simulink model "rev0BB"  (R2017b)
settings: Solver=FixedStepDiscrete  StartTime=0  StopTime=(((preLen+100+dataLenSymbols)*1+pad_first*3)*basePer)  RelTol=1e-3
values from neighbouring files (symbols this model uses):
  ack_stf_len_symbols = length(x_ACK_STF)    [rev0BB_setup.m]
  agc_delay_lag = 32    [rev0BB_setup.m]
  agc_detector_coef = ones(1,agc_detector_taps)./agc_detector_taps    [rev0BB_setup.m]
  agc_on = true    [rev0BB_startup.m]
  agc_sat_low = -agcSaturation    (= -12)    [rev0BB_setup.m]
  agc_sat_up = agcSaturation    (= 12)    [rev0BB_setup.m]
  agcDesired = 0    [rev0BB_setup.m]
  agcExpDomain = agcSaturation    (= 12)    [rev0BB_setup.m]
  agcExpResolution = 2^-5    (= 0.03125)    [rev0BB_setup.m]
  agcPwrAvgNum = 128    [rev0BB_setup.m]
  agcSaturation = 12    [rev0BB_setup.m]
  agcSettleThresh = 0.65    [rev0BB_setup.m]
  agcStep = 2^-8    (= 0.00390625)    [rev0BB_setup.m]
  atanDomain = 5    [rev0BB_setup.m]
  atanDomainTiming = 256    [rev0BB_setup.m]
  atanResolution = 2^-9    (= 0.001953125)    [rev0BB_setup.m]
  atanResolutionTiming = 2^-5    (= 0.03125)    [rev0BB_setup.m]
  averaging_num = ones(1, averaging_samples)    [rev0BB_setup.m]
  averaging_samples = 128    [rev0BB_setup.m]
  awgnSeed = abs(dBSnrRange(dBSnrInd)*1000+trial+10000000)    [plotBer.m]    (also in rev0BB_startup.m = 67)
  basePer = 1/baseFreq    (= 5e-08)    [rev0BB_setup.m]
  bitsPerSymbolHeader = log2(radixHeader)    [rev0BB_setup.m]
  bitsPerSymbolMax = log2(radixMax)    [rev0BB_setup.m]
  cal_sig_i_mult = 1.0    (= 1)    [rev0BB_startup.m]
  cal_sig_i_offset = 0.0    (= 0)    [rev0BB_startup.m]
  cal_sig_q_mult = 1.0    (= 1)    [rev0BB_startup.m]
  cal_sig_q_offset = 0.0    (= 0)    [rev0BB_startup.m]
  cefEarlyWarning = 256    [rev0BB_setup.m]
  cefLen = length(x_CEF)    [rev0BB_setup.m]
  channelFIR = zeros(1, round(maxSampleDelay)+1)    [rev0BB_startup.m]
  coarseCFOAdaptDelay = 1    [rev0BB_setup.m]
  cr_i = 0.020    (= 0.02)    [rev0BB_setup.m]
  cr_i_preamp = 2^-9    (= 0.001953125)    [rev0BB_setup.m]
  cr_int1_sat_low = -cr_integrator1_saturation    (= -0.6)    [rev0BB_setup.m]
  cr_int1_sat_up = cr_integrator1_saturation    (= 0.6)    [rev0BB_setup.m]
  cr_integrator1_decay = 1    [rev0BB_setup.m]
  cr_integrator1_saturation = 0.6    [rev0BB_setup.m]
  cr_mult_pipeline = 0    [rev0BB_setup.m]
  cr_p = 0.015    [rev0BB_setup.m]
  cr_sat2_low = -cr_saturation2    (= -0.6)    [rev0BB_setup.m]
  cr_sat2_up = cr_saturation2    (= 0.6)    [rev0BB_setup.m]
  cr_smooth_num = (1/cr_smooth_samples).*ones(1, cr_smooth_samples)    [rev0BB_setup.m]
  D_128 = [ 1,  8,  2,  4, 16, 32, 64]    [golay.m]    (also in rev0BB_setup.m)
  D_32 = [ 1,  4,  8,  2, 16]    [golay.m]    (also in rev0BB_setup.m)
  dataLenSymbols = header_len_bytes*8/bitsPerSymbolHeader + frame_len_bytes*8/bitsPerSymbol    [rev0BB_setup.m]
  default_channel = 3    [rev0BB_setup.m]
  dmm_coefs = ones(1,dmm_samples)./dmm_samples    [rev0BB_setup.m]
  dst_field_len = 8    [rev0BB_setup.m]
  expDomain = 3.3    [rev0BB_setup.m]
  expResolution = 2^-5    (= 0.03125)    [rev0BB_setup.m]
  expTol = .1    (= 0.1)    [rev0BB_setup.m]
  flush_delay = regular_pipeline*2+mult_pipeline+4    (= 4)    [rev0BB_setup.m]
  frac_lut_domain = 256    [rev0BB_setup.m]
  frac_lut_domain_cr = 64    [rev0BB_setup.m]
  frac_lut_range_max = 512    [rev0BB_setup.m]
  frac_lut_range_max_coarse_cfo = 127    [rev0BB_setup.m]
  frac_lut_range_max_cr = 127    [rev0BB_setup.m]
  frac_lut_range_min = -frac_lut_range_max    (= -512)    [rev0BB_setup.m]
  frac_lut_range_min_coarse_cfo = -frac_lut_range_max_coarse_cfo    (= -127)    [rev0BB_setup.m]
  frac_lut_range_min_cr = -frac_lut_range_max_cr    (= -127)    [rev0BB_setup.m]
  frac_lut_table_breaks = -frac_lut_domain:frac_lut_res:(frac_lut_domain-1)    [rev0BB_setup.m]
  frac_lut_table_breaks_coarse_cfo = -frac_lut_domain_coarse_cfo:frac_lut_res_coarse_cfo:(frac_lut_domain_coarse_cfo-1)    [rev0BB_setup.m]
  frac_lut_table_breaks_cr = -frac_lut_domain_cr:frac_lut_res_cr:(frac_lut_domain_cr-1)    [rev0BB_setup.m]
  frac_lut_table_data = 1./frac_lut_table_breaks    [rev0BB_setup.m]
  frac_lut_table_data_coarse_cfo = 1./frac_lut_table_breaks_coarse_cfo    [rev0BB_setup.m]
  frac_lut_table_data_cr = 1./frac_lut_table_breaks_cr    [rev0BB_setup.m]
  freeze_en_agc = true    [rev0BB_startup.m]
  freeze_en_cr_int1 = false    [rev0BB_startup.m]
  freeze_en_cr_int2 = false    [rev0BB_startup.m]
  freeze_en_cr_phase = false    [rev0BB_startup.m]
  freeze_en_tr_int1 = false    [rev0BB_startup.m]
  freeze_en_tr_int2 = false    [rev0BB_startup.m]
  freeze_en_tr_phase = false    [rev0BB_startup.m]
  freeze_on_cef_done = true    [rev0BB_startup.m]
  freeze_on_stf_done = false    [rev0BB_startup.m]
  freeze_on_valid = true    [rev0BB_startup.m]
  golay_type = 32    [rev0BB_setup.m]
  guardInt = int16(4)    [rev0BB_setup.m]
  guardTol = int16(5)    [rev0BB_setup.m]
  header_len_bytes = 8    [rev0BB_setup.m]
  lineWidth = 60    [rev0BB_setup.m]
  lmsEqDepth = 38    [rev0BB_setup.m]
  lmsStep_init = 0.006    [rev0BB_setup.m]
  lmsStep_meta = (lmsStep_final - lmsStep_init)/cefLen    [rev0BB_setup.m]
  lnDomain = 16    [rev0BB_setup.m]
  lnResolution = 2^-5    (= 0.03125)    [rev0BB_setup.m]
  local_node_id = 2    [rev0BB_startup.m]
  maxMsgSize = length(xSpectrum_PRE)+dataLenSymbols+300    [rev0BB_setup.m]
  minSTFPeaks = 3    [rev0BB_setup.m]
  mod_scheme_len_bytes = 1    [rev0BB_setup.m]
  modBPS = [1, 2, 4]    [rev0BB_setup.m]
  modKeys = [0, 1, 2]    [rev0BB_setup.m]
  mult_pipeline = 0    [rev0BB_setup.m]
  overSampleFreq = 80e6    (= 80000000)    [rev0BB_setup.m]
  overSamplePer = 1/overSampleFreq    (= 1.25e-08)    [rev0BB_setup.m]
  pad_first = 1000    [createTestVectors.m]
  post_cr_i_offset = 0    [rev0BB_startup.m]
  post_cr_q_offset = 0    [rev0BB_startup.m]
  preambleSequentialDetect = 2    [rev0BB_setup.m]
  preLen = length(x_PRE)    [rev0BB_setup.m]
  qam16_demod_scale_factor = qam16_hdl_distance/qam16_power_normalized_distance    [rev0BB_setup.m]
  rcRxFilt = [0.000303163120401141 -0.00118915940834234 -0.00187387637177 -0.00124167532697737 0.00029186889076529 0.00164526160586517 0.00182432050803312 0.000652133621739543 -0.00105668254004908 -0.00204011570659167 -0.00150058088768918 0.00026138356356816 0.0019831869994874 0.00231075800085521 0.000821993419120097 -0.00154687337975486 -0.00305430783933469 -0.00238186490079127 0.000301216962040692 0.00325307 ...(+2001 chars)    [rev0BB_setup.m]
  rcTxFilt = [0.000303163120401141 -0.00118915940834234 -0.00187387637177 -0.00124167532697737 0.00029186889076529 0.00164526160586517 0.00182432050803312 0.000652133621739543 -0.00105668254004908 -0.00204011570659167 -0.00150058088768918 0.00026138356356816 0.0019831869994874 0.00231075800085521 0.000821993419120097 -0.00154687337975486 -0.00305430783933469 -0.00238186490079127 0.000301216962040692 0.00325307 ...(+2001 chars)    [rev0BB_setup.m]
  regular_pipeline = 0    [rev0BB_setup.m]
  rx_gain = 1    [rev0BB_setup.m]
  rx_gain_i = 1    [rev0BB_setup.m]
  rx_gain_q = 1    [rev0BB_setup.m]
  rx_impare_i_offset = 0    [rev0BB_startup.m]
  rx_impare_i_scale = 1    [rev0BB_startup.m]
  rx_impare_q_offset = 0    [rev0BB_startup.m]
  rx_impare_q_scale = 1    [rev0BB_startup.m]
  rx_offset_correction_i = 0    [rev0BB_startup.m]
  rx_offset_correction_q = 0    [rev0BB_startup.m]
  sin_source_amp = 1    [rev0BB_setup.m]
  sin_source_freq = 250e6/16    (= 15625000)    [rev0BB_setup.m]
  slowPer = overSamplePer*slowSample    (= 2.5e-08)    [rev0BB_setup.m]
  std_pkt_type = 0    [rev0BB_setup.m]
  stfLen = length(x_STF)    [rev0BB_setup.m]
  testMsg = cat(1, xCTRL_PRE_adj, header, payload)    [plotBer.m]
  timing_i = 0.25    [rev0BB_setup.m]
  ... (+25 more)
undefined symbols (not defined in the file or in its folder): cr_integrator2_saturation, doppler, i, magnitude, useFadingChannel
libraries: helperLib x128, simulink x90, golayLib x34, dspsigops x32, commfilt2 x27, commdigbbndpm3 x8, hdlsllib x6, dsparch4 x4, commdigbbndam3 x4, commchan3 x2, commrflib2 x2, commcrc2 x2
(part 3 of 10)

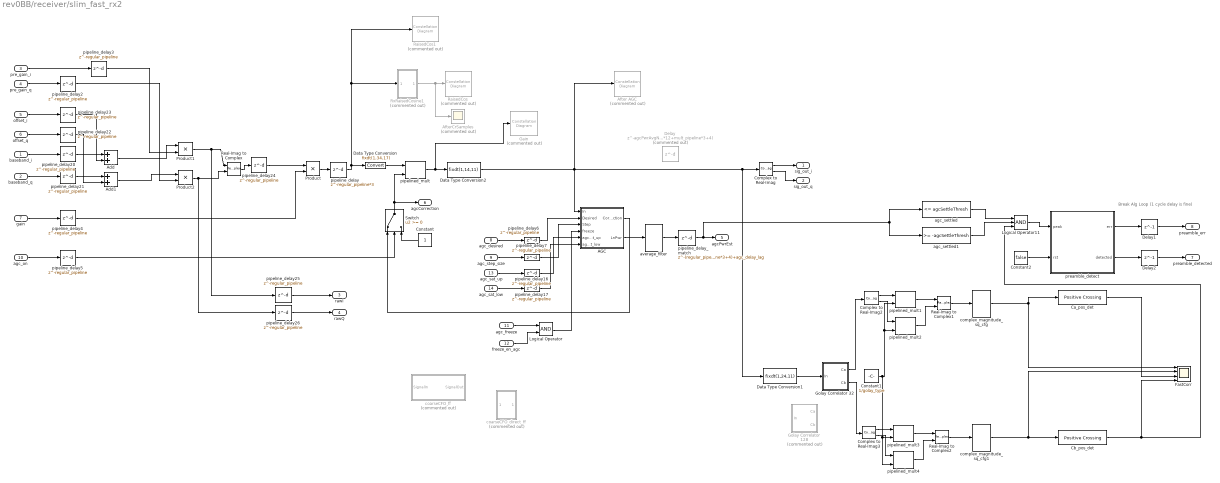
== system rev0BB/receiver/slim_fast_rx2 ==
  note: Break Alg Loop (1 cycle delay is fine)
  baseband_i : Inport
  baseband_q : Inport  Port=2
  pre_gain_i : Inport  Port=3
  pre_gain_q : Inport  Port=4
  offset_i : Inport  Port=5
  offset_q : Inport  Port=6
  gain : Inport  Port=7
  agc_desired : Inport  Port=8
  agc_step_size : Inport  Port=9
  agc_on : Inport  Port=10  OutDataTypeStr=boolean
  agc_freeze : Inport  Port=11  OutDataTypeStr=boolean
  freeze_en_agc : Inport  Port=12  OutDataTypeStr=boolean
  agc_sat_up : Inport  Port=13
  agc_sat_low : Inport  Port=14
  " RaisedCos" : ConstellationDiagram  Commented=on
  " RaisedCos1" : ConstellationDiagram  Commented=on
  AGC : Subsystem
  Add : Sum
  Add1 : Sum
  After AGC : ConstellationDiagram  Commented=on
  AfterCrSamples : Scope  Commented=on
  Ca_pos_det : helperLib/Positive Crossing  crossPt=trigger
  Cb_pos_det : helperLib/Positive Crossing  crossPt=trigger
  Complex to Real-Imag : ComplexToRealImag
  Complex to Real-Imag2 : ComplexToRealImag
  Complex to Real-Imag3 : ComplexToRealImag
  Constant : Constant  OutDataTypeStr=Inherit: Inherit via back propagation  SampleTime=-1
  Constant1 : Constant  Value=1/golay_type  OutDataTypeStr=Inherit: Inherit via back propagation
  Constant2 : Constant  Value=false  SampleTime=-1
  Data Type Conversion : DataTypeConversion  OutDataTypeStr=fixdt(1,34,17)
  Data Type Conversion1 : DataTypeConversion  OutDataTypeStr=fixdt(1,24,11)
  Data Type Conversion2 : DataTypeConversion  OutDataTypeStr=fixdt(1,14,11)
  Delay : Delay  Commented=on  DelayLength=agcPwrAvgNum/2-(regular_pipeline*12+mult_pipeline*3+4)  InitialCondition=0
  Delay1 : Delay  DelayLength=1  InitialCondition=0
  Delay2 : Delay  DelayLength=1  InitialCondition=0
  FastCorr : Scope  NumInputPorts=4
  Gain : ConstellationDiagram  Commented=on
  Golay Correlator 128 : Subsystem  Commented=on
  Golay Correlator 32 : Subsystem
  Logical Operator : Logic  AllPortsSameDT=off  OutDataTypeStr=boolean
  Logical Operator11 : Logic  Inputs=3  AllPortsSameDT=off  OutDataTypeStr=boolean
  Product : Product  OutDataTypeStr=Inherit: Same as first input
  Product1 : Product  OutDataTypeStr=Inherit: Same as first input
  Product2 : Product  OutDataTypeStr=Inherit: Same as first input
  Real-Imag to Complex : RealImagToComplex
  Real-Imag to Complex1 : RealImagToComplex
  Real-Imag to Complex2 : RealImagToComplex
  RxRaisedCosine1 : Subsystem  Commented=on
  Switch : Switch
  agc_settled : simulink/Logic and Bit Operations/Compare To Constant  relop=<=  const=agcSettleThresh  OutDataTypeStr=boolean
  agc_settled1 : simulink/Logic and Bit Operations/Compare To Constant  relop=>=  const=-agcSettleThresh  OutDataTypeStr=boolean
  average_filter : helperLib/average_filter  pipe=regular_pipeline  samples=agcPwrAvgNum  gain=1/agcPwrAvgNum
  coarseCFO_direct_ff : Subsystem  Commented=on
  coarseCFO_ff : Subsystem  Commented=on
  complex_magnitude_sq_cfg : helperLib/complex_magnitude_sq_cfg  mult=mult_pipeline  pipe=regular_pipeline
  complex_magnitude_sq_cfg1 : helperLib/complex_magnitude_sq_cfg  mult=mult_pipeline  pipe=regular_pipeline
  pipeline_delay : Delay  DelayLength=regular_pipeline*3
  pipeline_delay{2..7,16..17,20..26} (15 alike) : Delay  DelayLength=regular_pipeline
  pipeline_delay_match : Delay  DelayLength=(regular_pipeline*12+mult_pipeline*3+4)+agc_delay_lag
  pipelined_mult : helperLib/pipelined_mult  d=wide_mult_pipeline
  pipelined_mult{1..4} (4 alike) : helperLib/pipelined_mult  d=mult_pipeline
  preamble_detect : Stateflow chart  TreatAsAtomicUnit=on
  sig_out_i : Outport
  sig_out_q : Outport  Port=2
  rawI : Outport  Port=3
  rawQ : Outport  Port=4
  agcPwrEst : Outport  Port=5
  agcCorrection : Outport  Port=6
  preamble_detected : Outport  Port=7
  preamble_err : Outport  Port=8
  wires:
  agc_on/1 -> pipeline_delay5/1
  Add/1 -> Product1/1
  agc_freeze/1 -> Logical Operator/1
  pipeline_delay16/1 -> AGC/5(agc_sat_up)
  agc_sat_low/1 -> pipeline_delay17/1
  Data Type Conversion/1 -> pipelined_mult/1
  Switch/1 -> agcCorrection/1, pipelined_mult/2
  pipeline_delay4/1 -> Product/2
  gain/1 -> pipeline_delay4/1
  pre_gain_q/1 -> pipeline_delay2/1
  pre_gain_i/1 -> pipeline_delay3/1
  pipeline_delay20/1 -> Add/1
  Logical Operator/1 -> AGC/4(freeze)
  Real-Imag to Complex/1 -> pipeline_delay24/1
  pipeline_delay17/1 -> AGC/6(agc_sat_low)
  Add1/1 -> Product2/1
  agc_sat_up/1 -> pipeline_delay16/1
  pipeline_delay25/1 -> rawI/1
  agc_step_size/1 -> pipeline_delay7/1
  baseband_i/1 -> pipeline_delay20/1
  Product1/1 -> Real-Imag to Complex/1, pipeline_delay25/1
  pipeline_delay23/1 -> Add/2
  baseband_q/1 -> pipeline_delay21/1
  agc_desired/1 -> pipeline_delay6/1
  pipeline_delay6/1 -> AGC/2(Desired)
  pipeline_delay7/1 -> AGC/3(Step)
  Product2/1 -> Real-Imag to Complex/2, pipeline_delay26/1
  AGC/1(Correction) -> Switch/1
  pipeline_delay5/1 -> Switch/2
  pipeline_delay26/1 -> rawQ/1
  Constant/1 -> Switch/3
  RxRaisedCosine1/1(Out2) -> AfterCrSamples/1, " RaisedCos"/1
  AGC/2(LnPwr) -> average_filter/1
  pipeline_delay/1 -> Data Type Conversion/1, RxRaisedCosine1/1(In2), " RaisedCos1"/1
  pipeline_delay21/1 -> Add1/1
  freeze_en_agc/1 -> Logical Operator/2
  offset_q/1 -> pipeline_delay22/1
  pipeline_delay22/1 -> Add1/2
  pipelined_mult/1 -> Gain/1, Data Type Conversion2/1
  pipeline_delay24/1 -> Product/1
  Product/1 -> pipeline_delay/1
  Data Type Conversion2/1 -> After AGC/1, Data Type Conversion1/1, Complex to Real-Imag/1, AGC/1(In)
  offset_i/1 -> pipeline_delay23/1
  average_filter/1 -> pipeline_delay_match/1
  Complex to Real-Imag/1 -> sig_out_i/1
  Complex to Real-Imag/2 -> sig_out_q/1
  Complex to Real-Imag3/1 -> pipelined_mult3/1
  Golay Correlator 32/2(Cb) -> Complex to Real-Imag3/1
  complex_magnitude_sq_cfg/1 -> FastCorr/1, Ca_pos_det/1
  Complex to Real-Imag2/1 -> pipelined_mult1/1
  complex_magnitude_sq_cfg1/1 -> FastCorr/2, Cb_pos_det/1
  Golay Correlator 32/1(Ca) -> Complex to Real-Imag2/1
  Real-Imag to Complex2/1 -> complex_magnitude_sq_cfg1/1
  Real-Imag to Complex1/1 -> complex_magnitude_sq_cfg/1
  Data Type Conversion1/1 -> Golay Correlator 32/1(In)
  Complex to Real-Imag3/2 -> pipelined_mult4/1
  pipelined_mult4/1 -> Real-Imag to Complex2/2
  Constant1/1 -> pipelined_mult2/2, pipelined_mult1/2, pipelined_mult4/2, pipelined_mult3/2
  pipelined_mult2/1 -> Real-Imag to Complex1/2
  pipelined_mult1/1 -> Real-Imag to Complex1/1
  Complex to Real-Imag2/2 -> pipelined_mult2/1
  pipelined_mult3/1 -> Real-Imag to Complex2/1
  Ca_pos_det/1 -> FastCorr/3
  Cb_pos_det/1 -> Logical Operator11/3, FastCorr/4
  agc_settled1/1 -> Logical Operator11/2
  pipeline_delay_match/1 -> agc_settled/1, agc_settled1/1, agcPwrEst/1
  agc_settled/1 -> Logical Operator11/1
  Constant2/1 -> preamble_detect/2(rst)
  Logical Operator11/1 -> preamble_detect/1(peak)
  preamble_detect/1(err) -> Delay1/1
  preamble_detect/2(detected) -> Delay2/1
  Delay1/1 -> preamble_err/1
  Delay2/1 -> preamble_detected/1
  pipeline_delay2/1 -> Product2/2
  pipeline_delay3/1 -> Product1/2

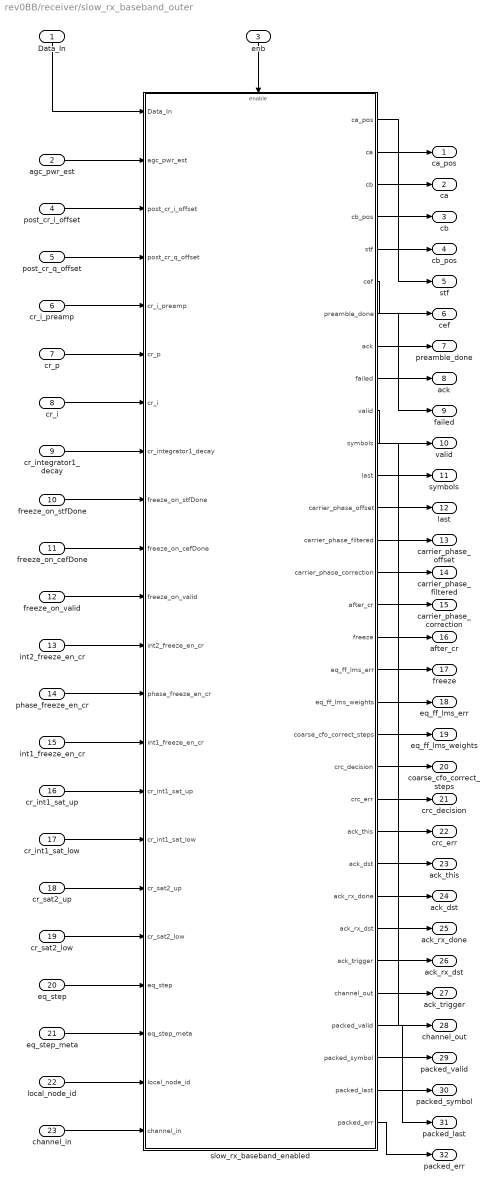
== system rev0BB/receiver/slow_rx_baseband_outer ==
  Data_In : Inport
  agc_pwr_est : Inport  Port=2  SampleTime=slowPer
  enb : Inport  Port=3
  post_cr_i_offset : Inport  Port=4
  post_cr_q_offset : Inport  Port=5
  cr_i_preamp : Inport  Port=6
  cr_p : Inport  Port=7
  cr_i : Inport  Port=8
  cr_integrator1_decay : Inport  Port=9
  freeze_on_stfDone : Inport  Port=10
  freeze_on_cefDone : Inport  Port=11
  freeze_on_valid : Inport  Port=12
  int2_freeze_en_cr : Inport  Port=13  OutDataTypeStr=boolean
  phase_freeze_en_cr : Inport  Port=14  OutDataTypeStr=boolean
  int1_freeze_en_cr : Inport  Port=15  OutDataTypeStr=boolean
  cr_int1_sat_up : Inport  Port=16
  cr_int1_sat_low : Inport  Port=17
  cr_sat2_up : Inport  Port=18
  cr_sat2_low : Inport  Port=19
  eq_step : Inport  Port=20
  eq_step_meta : Inport  Port=21
  local_node_id : Inport  Port=22
  channel_in : Inport  Port=23
  slow_rx_baseband_enabled : Subsystem
  ca_pos : Outport
  ca : Outport  Port=2
  cb : Outport  Port=3
  cb_pos : Outport  Port=4
  stf : Outport  Port=5
  cef : Outport  Port=6
  preamble_done : Outport  Port=7
  ack : Outport  Port=8
  failed : Outport  Port=9
  valid : Outport  Port=10
  symbols : Outport  Port=11
  last : Outport  Port=12
  carrier_phase_offset : Outport  Port=13
  carrier_phase_filtered : Outport  Port=14
  carrier_phase_correction : Outport  Port=15
  after_cr : Outport  Port=16
  freeze : Outport  Port=17  SampleTime=slowPer
  eq_ff_lms_err : Outport  Port=18  SampleTime=slowPer
  eq_ff_lms_weights : Outport  Port=19  SampleTime=slowPer
  coarse_cfo_correct_steps : Outport  Port=20  SampleTime=slowPer
  crc_decision : Outport  Port=21  SampleTime=slowPer
  crc_err : Outport  Port=22  SampleTime=slowPer
  ack_this : Outport  Port=23  SampleTime=slowPer
  ack_dst : Outport  Port=24  SampleTime=slowPer
  ack_rx_done : Outport  Port=25  SampleTime=slowPer
  ack_rx_dst : Outport  Port=26  SampleTime=slowPer
  ack_trigger : Outport  Port=27  SampleTime=slowPer
  channel_out : Outport  Port=28  SampleTime=slowPer
  packed_valid : Outport  Port=29  SampleTime=slowPer
  packed_symbol : Outport  Port=30  SampleTime=slowPer
  packed_last : Outport  Port=31  SampleTime=slowPer
  packed_err : Outport  Port=32  SampleTime=slowPer
  wires:
  slow_rx_baseband_enabled/1(ca_pos) -> ca_pos/1
  slow_rx_baseband_enabled/2(ca) -> ca/1
  slow_rx_baseband_enabled/3(cb) -> cb/1
  slow_rx_baseband_enabled/4(cb_pos) -> cb_pos/1
  slow_rx_baseband_enabled/5(stf) -> stf/1
  slow_rx_baseband_enabled/6(cef) -> cef/1
  slow_rx_baseband_enabled/7(preamble_done) -> preamble_done/1
  slow_rx_baseband_enabled/9(failed) -> failed/1
  slow_rx_baseband_enabled/10(valid) -> valid/1
  slow_rx_baseband_enabled/11(symbols) -> symbols/1
  slow_rx_baseband_enabled/13(carrier_phase_offset) -> carrier_phase_offset/1
  slow_rx_baseband_enabled/14(carrier_phase_filtered) -> carrier_phase_filtered/1
  slow_rx_baseband_enabled/15(carrier_phase_correction) -> carrier_phase_correction/1
  Data_In/1 -> slow_rx_baseband_enabled/1(Data_In)
  enb/1 -> slow_rx_baseband_enabled/Enable
  slow_rx_baseband_enabled/16(after_cr) -> after_cr/1
  post_cr_i_offset/1 -> slow_rx_baseband_enabled/3(post_cr_i_offset)
  post_cr_q_offset/1 -> slow_rx_baseband_enabled/4(post_cr_q_offset)
  cr_i_preamp/1 -> slow_rx_baseband_enabled/5(cr_i_preamp)
  cr_p/1 -> slow_rx_baseband_enabled/6(cr_p)
  cr_i/1 -> slow_rx_baseband_enabled/7(cr_i)
  cr_integrator1_decay/1 -> slow_rx_baseband_enabled/8(cr_integrator1_decay)
  freeze_on_stfDone/1 -> slow_rx_baseband_enabled/9(freeze_on_stfDone)
  freeze_on_cefDone/1 -> slow_rx_baseband_enabled/10(freeze_on_cefDone)
  freeze_on_valid/1 -> slow_rx_baseband_enabled/11(freeze_on_valid)
  slow_rx_baseband_enabled/17(freeze) -> freeze/1
  int2_freeze_en_cr/1 -> slow_rx_baseband_enabled/12(int2_freeze_en_cr)
  cr_int1_sat_up/1 -> slow_rx_baseband_enabled/15(cr_int1_sat_up)
  cr_int1_sat_low/1 -> slow_rx_baseband_enabled/16(cr_int1_sat_low)
  cr_sat2_up/1 -> slow_rx_baseband_enabled/17(cr_sat2_up)
  cr_sat2_low/1 -> slow_rx_baseband_enabled/18(cr_sat2_low)
  phase_freeze_en_cr/1 -> slow_rx_baseband_enabled/13(phase_freeze_en_cr)
  int1_freeze_en_cr/1 -> slow_rx_baseband_enabled/14(int1_freeze_en_cr)
  slow_rx_baseband_enabled/12(last) -> last/1
  slow_rx_baseband_enabled/18(eq_ff_lms_err) -> eq_ff_lms_err/1
  agc_pwr_est/1 -> slow_rx_baseband_enabled/2(agc_pwr_est)
  eq_step/1 -> slow_rx_baseband_enabled/19(eq_step)
  eq_step_meta/1 -> slow_rx_baseband_enabled/20(eq_step_meta)
  slow_rx_baseband_enabled/20(coarse_cfo_correct_steps) -> coarse_cfo_correct_steps/1
  slow_rx_baseband_enabled/19(eq_ff_lms_weights) -> eq_ff_lms_weights/1
  slow_rx_baseband_enabled/21(crc_decision) -> crc_decision/1
  slow_rx_baseband_enabled/22(crc_err) -> crc_err/1
  local_node_id/1 -> slow_rx_baseband_enabled/21(local_node_id)
  slow_rx_baseband_enabled/23(ack_this) -> ack_this/1
  slow_rx_baseband_enabled/24(ack_dst) -> ack_dst/1
  slow_rx_baseband_enabled/8(ack) -> ack/1
  slow_rx_baseband_enabled/25(ack_rx_done) -> ack_rx_done/1
  slow_rx_baseband_enabled/26(ack_rx_dst) -> ack_rx_dst/1
  slow_rx_baseband_enabled/27(ack_trigger) -> ack_trigger/1
  slow_rx_baseband_enabled/28(channel_out) -> channel_out/1
  channel_in/1 -> slow_rx_baseband_enabled/22(channel_in)
  slow_rx_baseband_enabled/29(packed_valid) -> packed_valid/1
  slow_rx_baseband_enabled/30(packed_symbol) -> packed_symbol/1
  slow_rx_baseband_enabled/31(packed_last) -> packed_last/1
  slow_rx_baseband_enabled/32(packed_err) -> packed_err/1

== system rev0BB/transmitter/transmitter_internal ==
  note: Logic for zero filling in upsample
  symbol : Inport  SampleTime=overSamplePer
  gain : Inport  Port=2  OutDataTypeStr=fixdt(1,8,4)  SampleTime=overSamplePer
  zero : Inport  Port=3  OutDataTypeStr=boolean  SampleTime=overSamplePer
  ModMode : Inport  Port=4  SampleTime=overSamplePer
  BPSK Modulator Baseband : commdigbbndpm3/BPSK Modulator Baseband  Ph=0  outDtype=Fixed-point  outWordLen=16  outUDDataType=sfix(16)  outFracLenMode=User-defined  outFracLen=13  outDataTypeStr=fixdt(1,16,13)  outLastDataTypeStr=fixdt(1,16,13)
  Compare To Zero : simulink/Logic and Bit Operations/Compare To Zero  relop=~=  OutDataTypeStr=boolean
  Complex to Real-Imag : ComplexToRealImag
  Constant : Constant  Value=0  OutDataTypeStr=fixdt(1,16,14)  SampleTime=-1
  Constant1 : Constant  Value=0  OutDataTypeStr=fixdt(1,16,14)  SampleTime=-1
  Constant2 : Constant  OutDataTypeStr=Inherit: Inherit via back propagation  SampleTime=-1
  Data Type Conversion : DataTypeConversion  OutDataTypeStr=uint32
  Data Type Conversion1 : DataTypeConversion  OutDataTypeStr=uint32
  Data Type Conversion2 : DataTypeConversion  OutDataTypeStr=uint32
  Data Type Conversion3 : DataTypeConversion  OutDataTypeStr=fixdt(1,24,19)
  Data Type Conversion4 : DataTypeConversion  OutDataTypeStr=fixdt(1,16,13)
  Data Type Conversion5 : DataTypeConversion  Commented=on  OutDataTypeStr=fixdt(1,28,23)
  Display : Display
  Extract Bits : simulink/Logic and Bit Operations/Extract Bits  bitsToExtract=Range of bits  numBits=8  bitIdxRange=[0 0]  outScalingMode=Preserve fixed-point scaling
      settings: SourceProductName=Simulink
  Extract Bits1 : simulink/Logic and Bit Operations/Extract Bits  bitsToExtract=Range of bits  numBits=8  bitIdxRange=[0 1]  outScalingMode=Preserve fixed-point scaling
      settings: SourceProductName=Simulink
  Extract Bits2 : simulink/Logic and Bit Operations/Extract Bits  bitsToExtract=Range of bits  numBits=8  bitIdxRange=[0 3]  outScalingMode=Preserve fixed-point scaling
      settings: SourceProductName=Simulink
  Gain : Gain  Gain=2  OutDataTypeStr=Inherit: Same as input
  Logical Operator : Logic  Operator=OR  AllPortsSameDT=off  OutDataTypeStr=boolean
  Multiport Switch : MultiPortSwitch
  Product : Product  OutDataTypeStr=Inherit: Same as first input
  QPSK Modulator Baseband : commdigbbndpm3/QPSK Modulator Baseband  InType=Integer  Enc=Gray  Ph=pi/4  outDtype=Fixed-point  outWordLen=16  outUDDataType=sfix(16)  outFracLenMode=User-defined  outFracLen=13  outDataTypeStr=fixdt(1,16,13)  outLastDataTypeStr=fixdt(1,16,13)
  Real-Imag to Complex : RealImagToComplex
  Rectangular QAM Modulator Baseband : commdigbbndam3/Rectangular QAM Modulator Baseband  M=16  InType=Integer  Enc=Gray  Mapping=[0:15]  PowType=Average Power  MinDist=2  AvgPow=1  PeakPow=1  Ph=0  outDtype=Fixed-point  outWordLen=16  outUDDataType=sfix(16)  outFracLenMode=User-defined  outFracLen=13  outDataTypeStr=fixdt(1,16,13)  outLastDataTypeStr=fixdt(1,16,13)
  Sum : Sum  Inputs=|++  OutDataTypeStr=Inherit: Same as first input
  Switch : Switch
  Tx_LPF : Subsystem
  mult_delay1 : Delay  DelayLength=mult_pipeline
  mult_delay2 : Delay  DelayLength=mult_pipeline
  pipeline_delay1 : Delay  DelayLength=regular_pipeline
  pipeline_delay3 : Delay  DelayLength=regular_pipeline
  raised_cosine : Subsystem
  zero_fill_counter : Subsystem
  baseband_i : Outport  SampleTime=overSamplePer  InitialOutput=[0]
  baseband_q : Outport  Port=2  SampleTime=overSamplePer  InitialOutput=[0]
  wires:
  symbol/1 -> Extract Bits1/1, Extract Bits2/1, Extract Bits/1
  Complex to Real-Imag/1 -> baseband_i/1
  Complex to Real-Imag/2 -> baseband_q/1
  Switch/1 -> Data Type Conversion3/1
  pipeline_delay1/1 -> raised_cosine/1(In1)
  Multiport Switch/1 -> Switch/3
  Gain/1 -> Data Type Conversion4/1
  Product/1 -> pipeline_delay3/1
  gain/1 -> mult_delay2/1
  mult_delay1/1 -> Product/1
  mult_delay2/1 -> Product/2
  pipeline_delay3/1 -> Complex to Real-Imag/1
  zero/1 -> Logical Operator/1
  Constant1/1 -> Real-Imag to Complex/2
  Constant/1 -> Real-Imag to Complex/1
  Real-Imag to Complex/1 -> Switch/1
  Logical Operator/1 -> Switch/2
  Compare To Zero/1 -> Logical Operator/2
  zero_fill_counter/1(Out1) -> Compare To Zero/1
  BPSK Modulator Baseband/1 -> Multiport Switch/2
  Rectangular QAM Modulator Baseband/1 -> Multiport Switch/4
  Extract Bits/1 -> Data Type Conversion/1
  Data Type Conversion/1 -> Display/1, BPSK Modulator Baseband/1
  Extract Bits1/1 -> Data Type Conversion1/1
  QPSK Modulator Baseband/1 -> Multiport Switch/3
  Extract Bits2/1 -> Data Type Conversion2/1
  ModMode/1 -> Sum/1
  Sum/1 -> Multiport Switch/1
  Constant2/1 -> Sum/2
  Data Type Conversion1/1 -> QPSK Modulator Baseband/1
  Data Type Conversion2/1 -> Rectangular QAM Modulator Baseband/1
  Data Type Conversion3/1 -> pipeline_delay1/1
  Data Type Conversion4/1 -> mult_delay1/1
  raised_cosine/1(Out1) -> Tx_LPF/1(In1)
  Tx_LPF/1(Out1) -> Gain/1

== system rev0BB/receiver/fast_rx_baseband/Timing Recovery ==
  note: It takes 13 cycles for the fractional delay to be seen
      | at the output of the farrow filter (after the pipeline delay).
  note: 12 cycles through farrow for new fractional delay to appear
  note: Error in Samples
  note: magnitude has delay
  note: This timing recovery block is based on the Mathworks Example and its primary reference, Digital Communication Receivers by Meyr. It particularly is based on pg 283 - 295, pg 291, pg 505-530, and 529-530
  uncorrected_oversampled : Inport
  timing_pre_scale : Inport  Port=2
  timing_p : Inport  Port=3
  timing_i : Inport  Port=4
  timing_integrator1_decay : Inport  Port=5
  int2_freeze : Inport  Port=6  OutDataTypeStr=boolean
  phase_freeze : Inport  Port=7  OutDataTypeStr=boolean
  int1_freeze : Inport  Port=8  OutDataTypeStr=boolean
  tr_int1_sat_up : Inport  Port=9
  tr_int1_sat_low : Inport  Port=10
  tr_sat2_up : Inport  Port=11
  tr_sat2_low : Inport  Port=12
  Compare To Zero : simulink/Logic and Bit Operations/Compare To Zero  relop=<=  OutDataTypeStr=boolean
  Constant1 : Constant  Value=0  OutDataTypeStr=Inherit: Inherit via back propagation  SampleTime=-1
  Constant2 : Constant  OutDataTypeStr=Inherit: Inherit via back propagation  SampleTime=-1
  Data Type Conversion : DataTypeConversion  OutDataTypeStr=single
  Delay : Delay  DelayLength=1  InitialCondition=0
  Delay1 : Delay  DelayLength=1  InitialCondition=0
  Delay12 : Delay  DelayLength=1
  SampleAccum : Subsystem
  Scope : Scope  Commented=on
  Subtract : Sum  Inputs=+-  OutDataTypeStr=Inherit: Same as first input
  Switch : Switch  Criteria=u2 > Threshold
  Switch1 : Switch  Criteria=u2 > Threshold
  Switch2 : Switch  Criteria=u2 > Threshold
  frac_delay_farrow_N-2_M-3 : Subsystem  AncestorBlock=helperLib/frac_delay_farrow_N-2_M-3  TreatAsAtomicUnit=on
  loopFilter : Subsystem
  nda_4x_time_err_enable : Subsystem  AncestorBlock=helperLib/nda_4x_time_err_enable  TreatAsAtomicUnit=on
  pipeline_delay2 : Delay  Commented=on  DelayLength=regular_pipeline
  pipeline_delay3 : Delay  DelayLength=regular_pipeline
  pipeline_delay5 : Delay  DelayLength=regular_pipeline
  pipeline_delay_match : Delay  DelayLength=3*mult_pipeline+regular_pipeline*(4-1)
  sat : Subsystem
  corrected_oversampled : Outport
  symbol_clock : Outport  Port=2
  timing_err : Outport  Port=3
  full_timing_delay : Outport  Port=4
  timing_raw_err : Outport  Port=5
  wires:
  Delay/1 -> Compare To Zero/1, Switch/3
  Switch/1 -> Subtract/1
  Constant2/1 -> Subtract/2
  Switch1/1 -> Switch2/3, Delay1/1, timing_err/1
  SampleAccum/2(clk_per) -> Switch/1
  Subtract/1 -> Delay/1
  uncorrected_oversampled/1 -> pipeline_delay5/1
  SampleAccum/3(fullDelay) -> full_timing_delay/1
  Data Type Conversion/1 -> nda_4x_time_err_enable/1(samples)
  Compare To Zero/1 -> SampleAccum/Enable, pipeline_delay_match/1, Switch/2
  SampleAccum/1(fracDelay) -> frac_delay_farrow_N-2_M-3/2(delay), Scope/1
  pipeline_delay5/1 -> frac_delay_farrow_N-2_M-3/1(samples)
  loopFilter/1(Out) -> Delay12/1
  frac_delay_farrow_N-2_M-3/1(out) -> pipeline_delay3/1
  pipeline_delay_match/1 -> symbol_clock/1, loopFilter/Enable, nda_4x_time_err_enable/2(enable)
  nda_4x_time_err_enable/1(err) -> sat/1(In1), timing_raw_err/1
  pipeline_delay3/1 -> corrected_oversampled/1, Data Type Conversion/1
  sat/1(Out1) -> loopFilter/1(In)
  timing_pre_scale/1 -> loopFilter/8(timing_pre_scale)
  timing_p/1 -> loopFilter/2(timing_p)
  timing_i/1 -> loopFilter/3(timing_i)
  timing_integrator1_decay/1 -> loopFilter/4(timing_integrator1_decay)
  pipeline_delay2/1 -> Switch1/3
  Delay1/1 -> Switch1/1
  int2_freeze/1 -> Switch1/2
  phase_freeze/1 -> Switch2/2
  Switch2/1 -> SampleAccum/1(correction)
  Constant1/1 -> Switch2/1
  tr_int1_sat_up/1 -> loopFilter/5(tr_int1_sat_up)
  tr_int1_sat_low/1 -> loopFilter/6(tr_int1_sat_low)
  int1_freeze/1 -> loopFilter/7(int1_freeze)
  tr_sat2_up/1 -> loopFilter/9(tr_sat2_up)
  tr_sat2_low/1 -> loopFilter/10(tr_sat2_low)
  Delay12/1 -> pipeline_delay2/1

== system rev0BB/receiver/slim_fast_rx/AGC ==
  note: Intentionally let width grow due to distinct chance of overflow
  In : Inport
  Desired : Inport  Port=2
  Step : Inport  Port=3
  freeze : Inport  Port=4  OutDataTypeStr=boolean
  agc_sat_up : Inport  Port=5
  agc_sat_low : Inport  Port=6
  Bit Shift : hdlsllib/Logic and Bit Operations/Bit Shift  Commented=on  mode=Shift Left Logical  N=1
      settings: SourceProductName=HDL Coder  SourceProductBaseCode=HD
  Constant : Constant  Value=0  OutDataTypeStr=Inherit: Inherit via back propagation  SampleTime=-1
  Data Type Duplicate : DataTypeDuplicate  Commented=on
  Data Type Duplicate1 : DataTypeDuplicate
  Data Type Conversion1 : DataTypeConversion  OutDataTypeStr=single
  Delay : Delay  DelayLength=1  InitialCondition=0
  Delay1 : Delay  DelayLength=1  InitialCondition=0
  Delay12 : Delay  DelayLength=1
  Discrete FIR Filter : DiscreteFir  FilterStructure=Direct form transposed  Coefficients=agc_detector_coef  InputProcessing=Columns as channels (frame based)  OutDataTypeStr=Inherit: Same as input
  Math Function : Math  SaturateOnIntegerOverflow=on
  Product : Product  Commented=on
  Saturation : Saturate  Commented=on  UpperLimit=agcSaturation  LowerLimit=-agcSaturation
  Saturation Dynamic : simulink/Discontinuities/Saturation Dynamic  OutMin=[]  OutMax=[]  OutDataTypeStr=Inherit: Same as second input  OutDataType=fixdt(1, 16)  OutScaling=2^-10  DoSatur=off
  Sum : Sum  Inputs=-+  OutDataTypeStr=Inherit: Same as first input
  Sum1 : Sum  Inputs=|++  OutDataTypeStr=Inherit: Same as first input
  Switch : Switch  Criteria=u2 > Threshold
  Switch1 : Switch  Criteria=u2 > Threshold
  complex_magnitude_sq_cfg : helperLib/complex_magnitude_sq_cfg  mult=wide_mult_pipeline  pipe=regular_pipeline
  exp : Subsystem  Commented=on
  exp1 : Subsystem  Commented=on
  ln1 : Subsystem
  mult_delay1 : Delay  Commented=on  DelayLength=wide_mult_pipeline
  pipeline_delay{,1..2,4,7..9,11..13} (10 alike) : Delay  DelayLength=regular_pipeline
  pipeline_delay10 : Delay  Commented=through  DelayLength=regular_pipeline
  pipeline_delay3 : Delay  Commented=on  DelayLength=regular_pipeline
  pipeline_delay5 : Delay  Commented=on  DelayLength=regular_pipeline
  pipeline_delay6 : Delay  DelayLength=regular_pipeline*2
  pipelined_mult2 : helperLib/pipelined_mult  d=wide_mult_pipeline
  Correction : Outport
  LnPwr : Outport  Port=2
  wires:
  In/1 -> Data Type Conversion1/1
  Data Type Conversion1/1 -> pipeline_delay6/1
  complex_magnitude_sq_cfg/1 -> pipeline_delay9/1
  ln1/1(Out) -> pipeline_delay10/1
  Sum/1 -> pipeline_delay/1
  pipeline_delay/1 -> pipelined_mult2/2
  pipeline_delay7/1 -> pipelined_mult2/1
  Bit Shift/1 -> pipeline_delay3/1
  Sum1/1 -> Delay/1
  exp1/1(Out) -> pipeline_delay5/1
  pipeline_delay5/1 -> Data Type Duplicate/2, Product/2
  Math Function/1 -> pipeline_delay4/1
  pipeline_delay4/1 -> Data Type Duplicate1/1, Correction/1
  Step/1 -> pipeline_delay7/1
  Desired/1 -> pipeline_delay8/1
  pipeline_delay10/1 -> Delay12/1
  pipeline_delay2/1 -> Math Function/1
  pipeline_delay3/1 -> exp1/1(In)
  pipeline_delay8/1 -> Sum/2
  pipeline_delay1/1 -> Data Type Duplicate1/2, ln1/2(data_type), Data Type Duplicate/1, Product/1, ln1/1(In)
  pipelined_mult2/1 -> Switch1/3
  Product/1 -> mult_delay1/1
  Switch/1 -> Bit Shift/1, pipeline_delay2/1, Delay1/1
  freeze/1 -> pipeline_delay13/1
  Delay1/1 -> Switch/1
  agc_sat_up/1 -> pipeline_delay11/1
  agc_sat_low/1 -> pipeline_delay12/1
  Delay/1 -> Saturation Dynamic/2
  pipeline_delay9/1 -> Discrete FIR Filter/1
  Discrete FIR Filter/1 -> pipeline_delay1/1
  pipeline_delay6/1 -> complex_magnitude_sq_cfg/1
  pipeline_delay13/1 -> Switch1/2, Switch/2
  Switch1/1 -> Sum1/1
  Constant/1 -> Switch1/1
  pipeline_delay12/1 -> Saturation Dynamic/3
  pipeline_delay11/1 -> Saturation Dynamic/1
  Saturation Dynamic/1 -> Sum1/2, Switch/3
  Delay12/1 -> LnPwr/1, Sum/1

== system rev0BB/receiver/slim_fast_rx/Golay Correlator 32 ==
  In : Inport
  GolayCoralatorBase_fp : golayLib/GolayCoralatorBase_fp  dSub=D_32(1)*4  wSub=W_32(1)  mult=0
  GolayCoralatorBase_fp1 : golayLib/GolayCoralatorBase_fp  dSub=D_32(2)*4  wSub=W_32(2)  mult=0
  GolayCoralatorBase_fp2 : golayLib/GolayCoralatorBase_fp  dSub=D_32(3)*4  wSub=W_32(3)  mult=0
  GolayCoralatorBase_fp3 : golayLib/GolayCoralatorBase_fp  dSub=D_32(4)*4  wSub=W_32(4)  mult=0
  GolayCoralatorBase_fp4 : golayLib/GolayCoralatorBase_fp  dSub=D_32(5)*4  wSub=W_32(5)  mult=0
  pipeline_delay{,1..13} (14 alike) : Delay  DelayLength=regular_pipeline
  Ca : Outport
  Cb : Outport  Port=2
  wires:
  GolayCoralatorBase_fp/1 -> pipeline_delay/1
  GolayCoralatorBase_fp/2 -> pipeline_delay1/1
  GolayCoralatorBase_fp1/1 -> pipeline_delay2/1
  GolayCoralatorBase_fp1/2 -> pipeline_delay3/1
  GolayCoralatorBase_fp4/1 -> pipeline_delay8/1
  GolayCoralatorBase_fp2/1 -> pipeline_delay4/1
  GolayCoralatorBase_fp2/2 -> pipeline_delay5/1
  GolayCoralatorBase_fp3/1 -> pipeline_delay6/1
  GolayCoralatorBase_fp3/2 -> pipeline_delay7/1
  pipeline_delay9/1 -> pipeline_delay11/1
  pipeline_delay8/1 -> pipeline_delay10/1
  pipeline_delay10/1 -> pipeline_delay12/1
  In/1 -> GolayCoralatorBase_fp/2, GolayCoralatorBase_fp/1
  pipeline_delay/1 -> GolayCoralatorBase_fp1/1
  pipeline_delay1/1 -> GolayCoralatorBase_fp1/2
  pipeline_delay2/1 -> GolayCoralatorBase_fp2/1
  pipeline_delay3/1 -> GolayCoralatorBase_fp2/2
  pipeline_delay4/1 -> GolayCoralatorBase_fp3/1
  pipeline_delay6/1 -> GolayCoralatorBase_fp4/1
  pipeline_delay12/1 -> Ca/1
  pipeline_delay13/1 -> Cb/1
  pipeline_delay5/1 -> GolayCoralatorBase_fp3/2
  pipeline_delay7/1 -> GolayCoralatorBase_fp4/2
  GolayCoralatorBase_fp4/2 -> pipeline_delay9/1
  pipeline_delay11/1 -> pipeline_delay13/1

== system rev0BB/receiver/slim_fast_rx/RxRaisedCosine2 ==
  note: Note: the tool should optomize a single FIR filter to this config due to 0 propogation. However, will make explicit for now
  note: (a+bj)(c+dj) = ac+adj+bcj-bd
      | If d = 0 | = ac + bcj
  note: Raised Cosine Filter Can be Split because it is Real (use 2 multiplies instead of 4 per tap)
  In2 : Inport
  Complex to Real-Imag : ComplexToRealImag
  Discrete FIR Filter : DiscreteFir  FilterStructure=Direct form transposed  Coefficients=rcRxFilt  AccumDataTypeStr=Inherit: Same as product output
  Discrete FIR Filter1 : DiscreteFir  FilterStructure=Direct form transposed  Coefficients=rcRxFilt  AccumDataTypeStr=Inherit: Same as product output
  Raised Cosine Receive Filter : commfilt2/Raised Cosine Receive Filter  Commented=on  filtType=Square root  R=.1  filtSpan=30  N=4  downFactor=1  downOffset=0  filterGain=1  InputProcessing=Columns as channels (frame based)  RateOptions=Enforce single-rate processing  framing=Mute  checkCoeff=on  variableName=rcRxFilt  currentFiltSpan=30  D=(30)/2  inputOffset=0  sampMode=Mute  saveAsFlag=0  rateMode=Downsampling  checkGain=Normalized  launchFVT=on  roundingMode=Floor  overflowMode=off  coeffDataTypeStr=Inherit: Same word length as input  coeffMin=[]  coeffMax=[]  coeffLastDataTypeStr=Inherit: Same word length as input  accumDataTypeStr=Inherit: Same as product output  accumLastDataTypeStr=Inherit: Same as product output  outputDataTypeStr=Inherit: Same as accumulator  outputMin=[]  outputMax=[]  outputLastDataTypeStr=Inherit: Same as accumulator
  Real-Imag to Complex : RealImagToComplex
  Out2 : Outport
  wires:
  In2/1 -> Complex to Real-Imag/1
  Complex to Real-Imag/1 -> Discrete FIR Filter/1
  Complex to Real-Imag/2 -> Discrete FIR Filter1/1
  Discrete FIR Filter/1 -> Real-Imag to Complex/1
  Discrete FIR Filter1/1 -> Real-Imag to Complex/2
  Real-Imag to Complex/1 -> Out2/1

== system rev0BB/receiver/slim_fast_rx/average_filter ==
  note: Clever Arch of an Averaging Filter I saw in A Split MAC Approach for SDR Platforms by Paolo Di Francesco, S´eamas McGettrick, Uchenna K. Anyanwu, James C. O’Sullivan,
      | Allen B. MacKenzie, and Luiz A. DaSilva.  This requires a shift register, 1 mult, and 2 adds (3 if you count the negation).  Downside is unpipelined loopback (standard IIR problem)
  In1 : Inport
  Data Type Conversion : DataTypeConversion
  Delay : Delay  DelayLength=samples  InitialCondition=0
  Delay1 : Delay  DelayLength=1  InitialCondition=0
  Gain : Gain  Gain=gain  OutDataTypeStr=Inherit: Same as input
  Sum : Sum  Inputs=|++  OutDataTypeStr=Inherit: Same as first input
  Sum1 : Sum  Inputs=|+-  OutDataTypeStr=Inherit: Same as first input
  pipeline_delay : Delay  DelayLength=pipe
  Out1 : Outport
  wires:
  Data Type Conversion/1 -> Sum/1
  pipeline_delay/1 -> Data Type Conversion/1, Delay/1
  Gain/1 -> pipeline_delay/1
  Delay1/1 -> Sum/2
  Sum1/1 -> Delay1/1, Out1/1
  Delay/1 -> Sum1/2
  In1/1 -> Gain/1
  Sum/1 -> Sum1/1

== system rev0BB/receiver/slim_fast_rx1/AGC ==
  note: Intentionally let width grow due to distinct chance of overflow
  In : Inport
  Desired : Inport  Port=2
  Step : Inport  Port=3
  freeze : Inport  Port=4  OutDataTypeStr=boolean
  agc_sat_up : Inport  Port=5
  agc_sat_low : Inport  Port=6
  Bit Shift : hdlsllib/Logic and Bit Operations/Bit Shift  Commented=on  mode=Shift Left Logical  N=1
      settings: SourceProductName=HDL Coder  SourceProductBaseCode=HD
  Constant : Constant  Value=0  OutDataTypeStr=Inherit: Inherit via back propagation  SampleTime=-1
  Data Type Duplicate : DataTypeDuplicate  Commented=on
  Data Type Duplicate1 : DataTypeDuplicate
  Data Type Conversion1 : DataTypeConversion  OutDataTypeStr=fixdt(1,38,18)
  Delay : Delay  DelayLength=1  InitialCondition=0
  Delay1 : Delay  DelayLength=1  InitialCondition=0
  Discrete FIR Filter : DiscreteFir  FilterStructure=Direct form transposed  Coefficients=agc_detector_coef  InputProcessing=Columns as channels (frame based)  OutDataTypeStr=Inherit: Same as input
  Product : Product  Commented=on
  Saturation : Saturate  Commented=on  UpperLimit=agcSaturation  LowerLimit=-agcSaturation
  Saturation Dynamic : simulink/Discontinuities/Saturation Dynamic  OutMin=[]  OutMax=[]  OutDataTypeStr=Inherit: Same as second input  OutDataType=fixdt(1, 16)  OutScaling=2^-10  DoSatur=off
  Sum : Sum  Inputs=-+
  Sum1 : Sum  Inputs=|++
  Switch : Switch  Criteria=u2 > Threshold
  Switch1 : Switch  Criteria=u2 > Threshold
  complex_magnitude_sq_cfg : helperLib/complex_magnitude_sq_cfg  mult=wide_mult_pipeline  pipe=regular_pipeline
  exp : Subsystem
  exp1 : Subsystem  Commented=on
  ln1 : Subsystem
  mult_delay1 : Delay  Commented=on  DelayLength=wide_mult_pipeline
  pipeline_delay{,1..2,4,7..13} (11 alike) : Delay  DelayLength=regular_pipeline
  pipeline_delay3 : Delay  Commented=on  DelayLength=regular_pipeline
  pipeline_delay5 : Delay  Commented=on  DelayLength=regular_pipeline
  pipeline_delay6 : Delay  DelayLength=regular_pipeline*2
  pipelined_mult2 : helperLib/pipelined_mult  d=wide_mult_pipeline
  Correction : Outport
  LnPwr : Outport  Port=2
  wires:
  In/1 -> Data Type Conversion1/1
  Data Type Conversion1/1 -> pipeline_delay6/1
  complex_magnitude_sq_cfg/1 -> pipeline_delay9/1
  ln1/1(Out) -> pipeline_delay10/1
  Sum/1 -> pipeline_delay/1
  pipeline_delay/1 -> pipelined_mult2/2
  pipeline_delay7/1 -> pipelined_mult2/1
  Bit Shift/1 -> pipeline_delay3/1
  Sum1/1 -> Delay/1
  exp1/1(Out) -> pipeline_delay5/1
  pipeline_delay5/1 -> Data Type Duplicate/2, Product/2
  exp/1(Out) -> pipeline_delay4/1
  pipeline_delay4/1 -> Data Type Duplicate1/1, Correction/1
  Step/1 -> pipeline_delay7/1
  Desired/1 -> pipeline_delay8/1
  pipeline_delay10/1 -> LnPwr/1, Sum/1
  pipeline_delay2/1 -> exp/1(In)
  pipeline_delay3/1 -> exp1/1(In)
  pipeline_delay8/1 -> Sum/2
  pipeline_delay1/1 -> Data Type Duplicate1/2, ln1/2(data_type), Data Type Duplicate/1, Product/1, ln1/1(In)
  Saturation Dynamic/1 -> Sum1/2, Switch/3
  pipelined_mult2/1 -> Switch1/3
  Product/1 -> mult_delay1/1
  Switch/1 -> Bit Shift/1, pipeline_delay2/1, Delay1/1
  freeze/1 -> pipeline_delay13/1
  Delay1/1 -> Switch/1
  agc_sat_up/1 -> pipeline_delay11/1
  agc_sat_low/1 -> pipeline_delay12/1
  Delay/1 -> Saturation Dynamic/2
  pipeline_delay9/1 -> Discrete FIR Filter/1
  Discrete FIR Filter/1 -> pipeline_delay1/1
  pipeline_delay6/1 -> complex_magnitude_sq_cfg/1
  pipeline_delay11/1 -> Saturation Dynamic/1
  pipeline_delay12/1 -> Saturation Dynamic/3
  pipeline_delay13/1 -> Switch1/2, Switch/2
  Switch1/1 -> Sum1/1
  Constant/1 -> Switch1/1

== system rev0BB/receiver/slim_fast_rx1/Golay Correlator 128 ==
  In : Inport
  GolayCoralatorBase_fp : golayLib/GolayCoralatorBase_fp  dSub=D_128(1)*4  wSub=W_128(1)  mult=0
  GolayCoralatorBase_fp1 : golayLib/GolayCoralatorBase_fp  dSub=D_128(2)*4  wSub=W_128(2)  mult=0
  GolayCoralatorBase_fp2 : golayLib/GolayCoralatorBase_fp  dSub=D_128(3)*4  wSub=W_128(3)  mult=0
  GolayCoralatorBase_fp3 : golayLib/GolayCoralatorBase_fp  dSub=D_128(4)*4  wSub=W_128(4)  mult=0
  GolayCoralatorBase_fp4 : golayLib/GolayCoralatorBase_fp  dSub=D_128(5)*4  wSub=W_128(5)  mult=0
  GolayCoralatorBase_fp5 : golayLib/GolayCoralatorBase_fp  dSub=D_128(6)*4  wSub=W_128(6)  mult=0
  GolayCoralatorBase_fp6 : golayLib/GolayCoralatorBase_fp  dSub=D_128(7)*4  wSub=W_128(7)  mult=0
  pipeline_delay{,1..13} (14 alike) : Delay  DelayLength=regular_pipeline
  Ca : Outport
  Cb : Outport  Port=2
  wires:
  GolayCoralatorBase_fp/1 -> pipeline_delay/1
  GolayCoralatorBase_fp/2 -> pipeline_delay1/1
  GolayCoralatorBase_fp1/1 -> pipeline_delay2/1
  GolayCoralatorBase_fp1/2 -> pipeline_delay3/1
  GolayCoralatorBase_fp4/1 -> pipeline_delay8/1
  GolayCoralatorBase_fp2/1 -> pipeline_delay4/1
  GolayCoralatorBase_fp2/2 -> pipeline_delay5/1
  GolayCoralatorBase_fp3/1 -> pipeline_delay6/1
  GolayCoralatorBase_fp3/2 -> pipeline_delay7/1
  GolayCoralatorBase_fp5/2 -> pipeline_delay11/1
  GolayCoralatorBase_fp5/1 -> pipeline_delay10/1
  GolayCoralatorBase_fp6/1 -> pipeline_delay12/1
  In/1 -> GolayCoralatorBase_fp/2, GolayCoralatorBase_fp/1
  pipeline_delay/1 -> GolayCoralatorBase_fp1/1
  pipeline_delay1/1 -> GolayCoralatorBase_fp1/2
  pipeline_delay2/1 -> GolayCoralatorBase_fp2/1
  pipeline_delay3/1 -> GolayCoralatorBase_fp2/2
  pipeline_delay4/1 -> GolayCoralatorBase_fp3/1
  pipeline_delay6/1 -> GolayCoralatorBase_fp4/1
  pipeline_delay8/1 -> GolayCoralatorBase_fp5/1
  pipeline_delay10/1 -> GolayCoralatorBase_fp6/1
  pipeline_delay12/1 -> Ca/1
  pipeline_delay13/1 -> Cb/1
  pipeline_delay5/1 -> GolayCoralatorBase_fp3/2
  pipeline_delay7/1 -> GolayCoralatorBase_fp4/2
  GolayCoralatorBase_fp4/2 -> pipeline_delay9/1
  pipeline_delay9/1 -> GolayCoralatorBase_fp5/2
  pipeline_delay11/1 -> GolayCoralatorBase_fp6/2
  GolayCoralatorBase_fp6/2 -> pipeline_delay13/1

== system rev0BB/receiver/slim_fast_rx1/Golay Correlator 32 ==
  In : Inport
  GolayCoralatorBase_fp : golayLib/GolayCoralatorBase_fp  dSub=D_32(1)*4  wSub=W_32(1)  mult=0
  GolayCoralatorBase_fp1 : golayLib/GolayCoralatorBase_fp  dSub=D_32(2)*4  wSub=W_32(2)  mult=0
  GolayCoralatorBase_fp2 : golayLib/GolayCoralatorBase_fp  dSub=D_32(3)*4  wSub=W_32(3)  mult=0
  GolayCoralatorBase_fp3 : golayLib/GolayCoralatorBase_fp  dSub=D_32(4)*4  wSub=W_32(4)  mult=0
  GolayCoralatorBase_fp4 : golayLib/GolayCoralatorBase_fp  dSub=D_32(5)*4  wSub=W_32(5)  mult=0
  pipeline_delay{,1..13} (14 alike) : Delay  DelayLength=regular_pipeline
  Ca : Outport
  Cb : Outport  Port=2
  wires:
  GolayCoralatorBase_fp/1 -> pipeline_delay/1
  GolayCoralatorBase_fp/2 -> pipeline_delay1/1
  GolayCoralatorBase_fp1/1 -> pipeline_delay2/1
  GolayCoralatorBase_fp1/2 -> pipeline_delay3/1
  GolayCoralatorBase_fp4/1 -> pipeline_delay8/1
  GolayCoralatorBase_fp2/1 -> pipeline_delay4/1
  GolayCoralatorBase_fp2/2 -> pipeline_delay5/1
  GolayCoralatorBase_fp3/1 -> pipeline_delay6/1
  GolayCoralatorBase_fp3/2 -> pipeline_delay7/1
  pipeline_delay9/1 -> pipeline_delay11/1
  pipeline_delay8/1 -> pipeline_delay10/1
  pipeline_delay10/1 -> pipeline_delay12/1
  In/1 -> GolayCoralatorBase_fp/2, GolayCoralatorBase_fp/1
  pipeline_delay/1 -> GolayCoralatorBase_fp1/1
  pipeline_delay1/1 -> GolayCoralatorBase_fp1/2
  pipeline_delay2/1 -> GolayCoralatorBase_fp2/1
  pipeline_delay3/1 -> GolayCoralatorBase_fp2/2
  pipeline_delay4/1 -> GolayCoralatorBase_fp3/1
  pipeline_delay6/1 -> GolayCoralatorBase_fp4/1
  pipeline_delay12/1 -> Ca/1
  pipeline_delay13/1 -> Cb/1
  pipeline_delay5/1 -> GolayCoralatorBase_fp3/2
  pipeline_delay7/1 -> GolayCoralatorBase_fp4/2
  GolayCoralatorBase_fp4/2 -> pipeline_delay9/1
  pipeline_delay11/1 -> pipeline_delay13/1

== system rev0BB/receiver/slim_fast_rx1/RxRaisedCosine1 ==
  In2 : Inport
  Discrete FIR Filter : DiscreteFir  FilterStructure=Direct form transposed  Coefficients=rcRxFilt  AccumDataTypeStr=Inherit: Same as product output
  Raised Cosine Receive Filter : commfilt2/Raised Cosine Receive Filter  Commented=on  filtType=Square root  R=0.2  filtSpan=10  N=4  downFactor=1  downOffset=0  filterGain=1  InputProcessing=Columns as channels (frame based)  RateOptions=Enforce single-rate processing  framing=Mute  checkCoeff=on  variableName=rcRxFilt  currentFiltSpan=10  D=5  inputOffset=0  sampMode=Mute  saveAsFlag=0  rateMode=Downsampling  checkGain=Normalized  launchFVT=on  roundingMode=Floor  overflowMode=off  coeffDataTypeStr=Inherit: Same word length as input  coeffMin=[]  coeffMax=[]  coeffLastDataTypeStr=Inherit: Same word length as input  accumDataTypeStr=Inherit: Same as product output  accumLastDataTypeStr=Inherit: Same as product output  outputDataTypeStr=Inherit: Same as accumulator  outputMin=[]  outputMax=[]  outputLastDataTypeStr=Inherit: Same as accumulator
  Out2 : Outport
  wires:
  Discrete FIR Filter/1 -> Out2/1
  In2/1 -> Discrete FIR Filter/1
